simulink model "text28"  (R2014a)
settings: Solver=FixedStepDiscrete  StartTime=0.0  StopTime=10.0  FixedStep=0.0005  RelTol=1e-3
libraries: simulink x70, ec55xxlib x61
(part 3 of 3)

== system text28/驱动系统/驱动逻辑/油门规则/油门刹车冲突 ==
  油门 : Inport
  刹车 : Inport  Port=2
  反馈 : Inport  Port=3
  If : If  NumInputs=2  IfExpression=u1>25&u2==1
  Merge2 : Merge
  故障 : Subsystem  TreatAsAtomicUnit=on
  "正常  " : Subsystem  TreatAsAtomicUnit=on
  Out1 : Outport
  wires:
  If/1 -> 故障/Action
  If/2 -> "正常  "/Action
  故障/1(Out1) -> Merge2/1
  Merge2/1 -> Out1/1
  "正常  "/1(Out1) -> Merge2/2
  反馈/1 -> "正常  "/1(In1)
  油门/1 -> If/1
  刹车/1 -> If/2

== system text28/驱动系统/驱动逻辑/油门规则/油门死区判断 ==
  In1 : Inport
  If1 : If  IfExpression=u1<5
  Merge : Merge
  油门大于5% : Subsystem  TreatAsAtomicUnit=on
  油门小于5% : Subsystem  TreatAsAtomicUnit=on
  Out1 : Outport
  wires:
  If1/1 -> 油门小于5%/Action
  If1/2 -> 油门大于5%/Action
  油门小于5%/1(Out1) -> Merge/1
  油门大于5%/1(Out1) -> Merge/2
  Merge/1 -> Out1/1
  In1/1 -> If1/1

== system text28/驱动系统/驱动逻辑/电机测速/Function-Call Subsystem4 ==
  In3 : Inport
  In1 : Inport  Port=2
  In2 : Inport  Port=3
  In4 : Inport  Port=4
  function : TriggerPort  TriggerType=function-call
  Terminator1 : Terminator
  Terminator2 : Terminator
  Terminator3 : Terminator
  "Out2 " : Outport
  wires:
  In3/1 -> Terminator2/1
  In1/1 -> Terminator1/1
  In2/1 -> "Out2 "/1
  In4/1 -> Terminator3/1

== system text28/驱动系统/驱动逻辑/电机测速/ReceiveMessages ==
  resive : Inport
  Active_Discharge_Enab_Ter : Terminator
  Data Type Conversion : DataTypeConversion
  Data Type Conversion1 : DataTypeConversion
  Gain : Gain  Gain=-1
  Gain1 : Gain  Gain=-1
  IGBT_Enable_Feedback_Ter : Terminator
  Livecounter_Ter : Terminator
  MeaModule : ec55xxlib/RapidECU_U2/11Calibration/MeaModule  signal=motor_speed
  MeaModule1 : ec55xxlib/RapidECU_U2/11Calibration/MeaModule  signal=motor_torque
  MotorACCurrent_Ter : Terminator
  Precharge_Allow_Ter : Terminator
  resive1 : Subsystem
  电机转速 : Outport
  电机扭矩 : Outport  Port=2
  wires:
  resive1/1(Precharge_Allow_Out) -> Precharge_Allow_Ter/1
  resive1/3(MotorACCurrent_Out) -> MotorACCurrent_Ter/1
  resive1/5(Livecounter_Out) -> Livecounter_Ter/1
  resive1/6(IGBT_Enable_Feedback_Out) -> IGBT_Enable_Feedback_Ter/1
  resive1/7(Active_Discharge_Enab_Out) -> Active_Discharge_Enab_Ter/1
  resive/1 -> resive1/1(input)
  MeaModule/1 -> 电机转速/1
  MeaModule1/1 -> 电机扭矩/1
  Gain/1 -> MeaModule/1
  resive1/4(Motor_Speed_Out) -> Data Type Conversion/1
  Data Type Conversion/1 -> Gain/1
  Gain1/1 -> MeaModule1/1
  resive1/2(MotorTorque_Out) -> Data Type Conversion1/1
  Data Type Conversion1/1 -> Gain1/1

== system text28/驱动系统/驱动逻辑/角度传感器/角度传感器数据处理及不可靠信号 ==
  角度1 : Inport
  角度2 : Inport  Port=2
  Abs : Abs
  Constant : Constant  Value=100
  MeaModule : ec55xxlib/RapidECU_U2/11Calibration/MeaModule  signal=apps_erro
  MeaModule1 : ec55xxlib/RapidECU_U2/11Calibration/MeaModule  signal=app_date1
  MeaModule3 : ec55xxlib/RapidECU_U2/11Calibration/MeaModule  signal=baifenbi3
  Product : Product
  Product1 : Product
  不可靠信号判断 : Subsystem
  油门数值处理 : Subsystem
  百分比转化 : Subsystem
  油门数值 : Outport
  油门百分比 : Outport  Port=2
  wires:
  Product/1 -> 油门数值/1
  角度2/1 -> 百分比转化/2(角度2), 油门数值处理/2(角度2)
  不可靠信号判断/1(Out1) -> MeaModule/1
  油门数值处理/1(油门数值) -> MeaModule1/1
  MeaModule/1 -> Product/2
  MeaModule1/1 -> Product/1
  百分比转化/1(Out2) -> Abs/1
  油门数值处理/2(油门百分比) -> 油门百分比/1
  角度1/1 -> 油门数值处理/1(角度1), 百分比转化/1(角度1)
  Abs/1 -> MeaModule3/1
  Constant/1 -> Product1/2
  Product1/1 -> 不可靠信号判断/1(In1)
  MeaModule3/1 -> Product1/1

== system text28/驱动系统/驱动逻辑/角度传感器/角度传感器是否正常 ==
  角度1 : Inport
  角度2 : Inport  Port=2
  If : If  NumInputs=2  IfExpression=u2 > 800 & u1>600 &u2 <2900&u1<2700
  If Action Subsystem : Subsystem  TreatAsAtomicUnit=on
  If Action Subsystem1 : Subsystem  TreatAsAtomicUnit=on
  Merge : Merge
  油门范围 : Outport
  wires:
  角度1/1 -> If/1
  If/1 -> If Action Subsystem1/Action
  If/2 -> If Action Subsystem/Action
  If Action Subsystem1/1(Out1) -> Merge/1
  If Action Subsystem/1(Out1) -> Merge/2
  Merge/1 -> 油门范围/1
  角度2/1 -> If/2

== system text28/驱动系统/驱动逻辑/制动与待驶/待驶激活/If Action Subsystem ==
  Action Port : ActionPort  ActionType=then
  Constant : Constant
  Out1 : Outport
  wires:
  Constant/1 -> Out1/1

== system text28/驱动系统/驱动逻辑/制动与待驶/待驶激活/If Action Subsystem1 ==
  Action Port : ActionPort  ActionType=else
  Constant : Constant  Value=0
  Out1 : Outport
  wires:
  Constant/1 -> Out1/1

== system text28/驱动系统/驱动逻辑/制动与待驶/待驶激活/If Action Subsystem2 ==
  Action Port : ActionPort  ActionType=then
  Constant : Constant
  Out1 : Outport
  wires:
  Constant/1 -> Out1/1

== system text28/驱动系统/驱动逻辑/制动与待驶/待驶激活/If Action Subsystem3 ==
  Action Port : ActionPort  ActionType=else
  Constant : Constant  Value=0
  Out1 : Outport
  wires:
  Constant/1 -> Out1/1

== system text28/驱动系统/驱动逻辑/制动与待驶/鸣笛1/If Action Subsystem ==
  Action Port : ActionPort  ActionType=then
  Constant2 : Constant
  Out1 : Outport
  wires:
  Constant2/1 -> Out1/1

== system text28/驱动系统/驱动逻辑/制动与待驶/鸣笛1/If Action Subsystem1 ==
  Action Port : ActionPort  ActionType=else
  Constant : Constant  Value=0
  Out1 : Outport
  wires:
  Constant/1 -> Out1/1

== system text28/驱动系统/驱动逻辑/制动与待驶/鸣笛1/鸣笛 ==
  In1 : Inport
  安全回路 : Inport  Port=2
  Constant3 : Constant
  Data Type Conversion : DataTypeConversion  OutDataTypeStr=uint32
  Data Type Conversion1 : DataTypeConversion  OutDataTypeStr=uint32
  If : If  IfExpression=u1>0&u1<150
  If Action Subsystem : Subsystem  TreatAsAtomicUnit=on
  If Action Subsystem1 : Subsystem  TreatAsAtomicUnit=on
  Merge : Merge
  Product : Product
  Sum : Sum  Inputs=|++
  Unit Delay : UnitDelay  SampleTime=-1
  蜂鸣器 : ec55xxlib/RapidECU_U2/06PowerDriverPWM/PowerDriverPWM  channel=117: O_PWM11_HS2A9  sampletime=-1
  wires:
  If/1 -> If Action Subsystem/Action
  Data Type Conversion/1 -> 蜂鸣器/1
  In1/1 -> Sum/1
  Data Type Conversion1/1 -> 蜂鸣器/2
  Constant3/1 -> Data Type Conversion/1
  If/2 -> If Action Subsystem1/Action
  Merge/1 -> Data Type Conversion1/1
  Product/1 -> Unit Delay/1, If/1
  Unit Delay/1 -> Sum/2
  If Action Subsystem/1(Out1) -> Merge/1
  If Action Subsystem1/1(Out1) -> Merge/2
  安全回路/1 -> Product/1
  Sum/1 -> Product/2

== system text28/驱动系统/驱动逻辑/油门规则/刹车判断/有刹车 ==
  Action Port : ActionPort  ActionType=else
  Constant : Constant  Value=0
  Out1 : Outport
  wires:
  Constant/1 -> Out1/1

== system text28/驱动系统/驱动逻辑/油门规则/刹车判断/没刹车 ==
  Action Port : ActionPort  ActionType=then
  Constant : Constant
  Out1 : Outport
  wires:
  Constant/1 -> Out1/1

== system text28/驱动系统/驱动逻辑/油门规则/动力允许判断/动力信号 ==
  Action Port : ActionPort  ActionType=then
  Constant : Constant
  Out1 : Outport
  wires:
  Constant/1 -> Out1/1

== system text28/驱动系统/驱动逻辑/油门规则/动力允许判断/故障信号 ==
  Action Port : ActionPort  ActionType=else
  Constant : Constant  Value=0
  Out1 : Outport
  wires:
  Constant/1 -> Out1/1

== system text28/驱动系统/驱动逻辑/油门规则/油门刹车冲突/故障 ==
  Action Port : ActionPort  ActionType=then
  Constant : Constant  Value=0
  Out1 : Outport
  wires:
  Constant/1 -> Out1/1

== system text28/驱动系统/驱动逻辑/油门规则/油门刹车冲突/正常   ==
  In1 : Inport
  Action Port : ActionPort  ActionType=else
  If : If  IfExpression=u1>=1
  Merge : Merge
  故障 : Subsystem  TreatAsAtomicUnit=on
  正常 : Subsystem  TreatAsAtomicUnit=on
  Out1 : Outport
  wires:
  In1/1 -> If/1
  If/1 -> 正常/Action
  If/2 -> 故障/Action
  正常/1(Out1) -> Merge/1
  故障/1(Out1) -> Merge/2
  Merge/1 -> Out1/1

== system text28/驱动系统/驱动逻辑/油门规则/油门死区判断/油门大于5% ==
  Action Port : ActionPort  ActionType=else
  Constant : Constant  Value=0
  Out1 : Outport
  wires:
  Constant/1 -> Out1/1

== system text28/驱动系统/驱动逻辑/油门规则/油门死区判断/油门小于5% ==
  Action Port : ActionPort  ActionType=then
  Constant : Constant
  Out1 : Outport
  wires:
  Constant/1 -> Out1/1

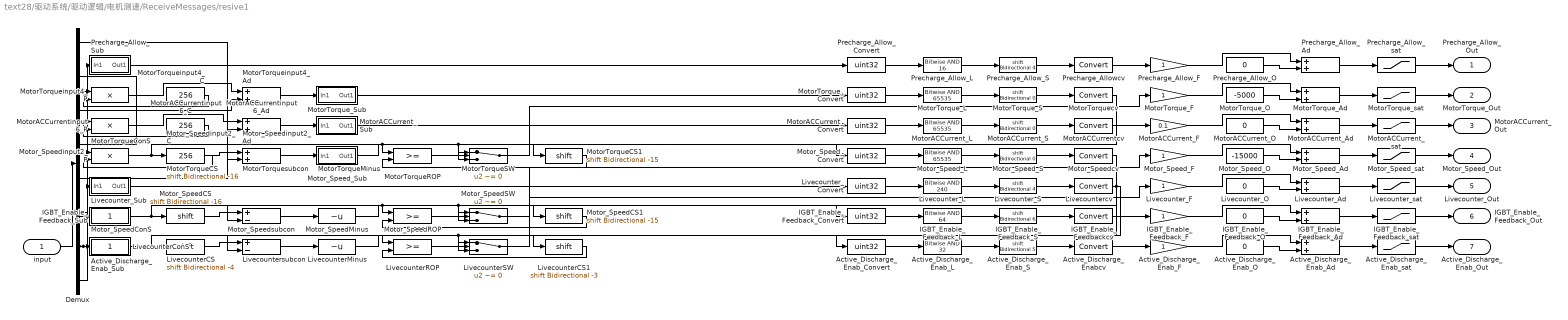
== system text28/驱动系统/驱动逻辑/电机测速/ReceiveMessages/resive1 ==
  input : Inport
  Active_Discharge_Enab_Ad : Sum
  Active_Discharge_Enab_Convert : DataTypeConversion  OutDataTypeStr=uint32
  Active_Discharge_Enab_F : Gain
  Active_Discharge_Enab_L : simulink/Logic and Bit Operations/Bitwise Operator  logicop=AND  UseBitMask=on  BitMask=32  BitMaskRealWorld=Stored Integer
  Active_Discharge_Enab_O : Constant  Value=0  OutDataTypeStr=single
  Active_Discharge_Enab_S : ArithShift  BitShiftNumber=5
  Active_Discharge_Enab_Sub : Subsystem
  Active_Discharge_Enab_sat : Saturate  UpperLimit=1  LowerLimit=0
  Active_Discharge_Enabcv : DataTypeConversion
  Demux : Demux  Outputs=8
  IGBT_Enable_Feedback_Ad : Sum
  IGBT_Enable_Feedback_Convert : DataTypeConversion  OutDataTypeStr=uint32
  IGBT_Enable_Feedback_F : Gain
  IGBT_Enable_Feedback_L : simulink/Logic and Bit Operations/Bitwise Operator  logicop=AND  UseBitMask=on  BitMask=64  BitMaskRealWorld=Stored Integer
  IGBT_Enable_Feedback_O : Constant  Value=0  OutDataTypeStr=single
  IGBT_Enable_Feedback_S : ArithShift  BitShiftNumber=6
  IGBT_Enable_Feedback_Sub : Subsystem
  IGBT_Enable_Feedback_sat : Saturate  UpperLimit=1  LowerLimit=0
  IGBT_Enable_Feedbackcv : DataTypeConversion
  LivecounterCS : ArithShift  BitShiftNumber=-4
  LivecounterCS1 : ArithShift  BitShiftNumber=-3
  LivecounterConS : Constant  OutDataTypeStr=single
  LivecounterMinus : UnaryMinus
  LivecounterROP : RelationalOperator  OutDataTypeStr=boolean
  LivecounterSW : Switch  Criteria=u2 ~= 0
  Livecounter_Ad : Sum
  Livecounter_Convert : DataTypeConversion  OutDataTypeStr=uint32
  Livecounter_F : Gain
  Livecounter_L : simulink/Logic and Bit Operations/Bitwise Operator  logicop=AND  UseBitMask=on  BitMask=240  BitMaskRealWorld=Stored Integer
  Livecounter_O : Constant  Value=0  OutDataTypeStr=single
  Livecounter_S : ArithShift  BitShiftNumber=4
  Livecounter_Sub : Subsystem
  Livecounter_sat : Saturate  UpperLimit=15  LowerLimit=0
  Livecountercv : DataTypeConversion
  Livecountersubcon : Sum  Inputs=+-
  MotorACCurrent_Ad : Sum
  MotorACCurrent_Convert : DataTypeConversion  OutDataTypeStr=uint32
  MotorACCurrent_F : Gain  Gain=0.1
  MotorACCurrent_L : simulink/Logic and Bit Operations/Bitwise Operator  logicop=AND  UseBitMask=on  BitMask=65535  BitMaskRealWorld=Stored Integer
  MotorACCurrent_O : Constant  Value=0  OutDataTypeStr=single
  MotorACCurrent_S : ArithShift
  MotorACCurrent_Sub : Subsystem
  MotorACCurrent_sat : Saturate  UpperLimit=1000  LowerLimit=0
  MotorACCurrentcv : DataTypeConversion
  MotorACCurrentinput6_Ad : Sum
  MotorACCurrentinput6_C : Constant  Value=256
  MotorACCurrentinput6_P : Product
  MotorTorqueCS : ArithShift  BitShiftNumber=-16
  MotorTorqueCS1 : ArithShift  BitShiftNumber=-15
  MotorTorqueConS : Constant  OutDataTypeStr=single
  MotorTorqueMinus : UnaryMinus
  MotorTorqueROP : RelationalOperator  OutDataTypeStr=boolean
  MotorTorqueSW : Switch  Criteria=u2 ~= 0
  MotorTorque_Ad : Sum
  MotorTorque_Convert : DataTypeConversion  OutDataTypeStr=uint32
  MotorTorque_F : Gain
  MotorTorque_L : simulink/Logic and Bit Operations/Bitwise Operator  logicop=AND  UseBitMask=on  BitMask=65535  BitMaskRealWorld=Stored Integer
  MotorTorque_O : Constant  Value=-5000  OutDataTypeStr=single
  MotorTorque_S : ArithShift
  MotorTorque_Sub : Subsystem
  MotorTorque_sat : Saturate  UpperLimit=5000  LowerLimit=-5000
  MotorTorquecv : DataTypeConversion
  MotorTorqueinput4_Ad : Sum
  MotorTorqueinput4_C : Constant  Value=256
  MotorTorqueinput4_P : Product
  MotorTorquesubcon : Sum  Inputs=+-
  Motor_SpeedCS : ArithShift  BitShiftNumber=-16
  Motor_SpeedCS1 : ArithShift  BitShiftNumber=-15
  Motor_SpeedConS : Constant  OutDataTypeStr=single
  Motor_SpeedMinus : UnaryMinus
  Motor_SpeedROP : RelationalOperator  OutDataTypeStr=boolean
  Motor_SpeedSW : Switch  Criteria=u2 ~= 0
  Motor_Speed_Ad : Sum
  Motor_Speed_Convert : DataTypeConversion  OutDataTypeStr=uint32
  Motor_Speed_F : Gain
  Motor_Speed_L : simulink/Logic and Bit Operations/Bitwise Operator  logicop=AND  UseBitMask=on  BitMask=65535  BitMaskRealWorld=Stored Integer
  Motor_Speed_O : Constant  Value=-15000  OutDataTypeStr=single
  Motor_Speed_S : ArithShift
  Motor_Speed_Sub : Subsystem
  Motor_Speed_sat : Saturate  UpperLimit=15000  LowerLimit=-15000
  Motor_Speedcv : DataTypeConversion
  Motor_Speedinput2_Ad : Sum
  Motor_Speedinput2_C : Constant  Value=256
  Motor_Speedinput2_P : Product
  Motor_Speedsubcon : Sum  Inputs=+-
  Precharge_Allow_Ad : Sum
  Precharge_Allow_Convert : DataTypeConversion  OutDataTypeStr=uint32
  Precharge_Allow_F : Gain
  Precharge_Allow_L : simulink/Logic and Bit Operations/Bitwise Operator  logicop=AND  UseBitMask=on  BitMask=16  BitMaskRealWorld=Stored Integer
  Precharge_Allow_O : Constant  Value=0  OutDataTypeStr=single
  Precharge_Allow_S : ArithShift  BitShiftNumber=4
  Precharge_Allow_Sub : Subsystem
  Precharge_Allow_sat : Saturate  UpperLimit=1  LowerLimit=0
  Precharge_Allowcv : DataTypeConversion
  Precharge_Allow_Out : Outport
  MotorTorque_Out : Outport  Port=2
  MotorACCurrent_Out : Outport  Port=3
  Motor_Speed_Out : Outport  Port=4
  Livecounter_Out : Outport  Port=5
  IGBT_Enable_Feedback_Out : Outport  Port=6
  Active_Discharge_Enab_Out : Outport  Port=7
  wires:
  Precharge_Allow_F/1 -> Precharge_Allow_Ad/1
  Precharge_Allow_O/1 -> Precharge_Allow_Ad/2
  Precharge_Allow_Ad/1 -> Precharge_Allow_sat/1
  Precharge_Allow_sat/1 -> Precharge_Allow_Out/1
  Demux/7 -> IGBT_Enable_Feedback_Sub/1(In1), Active_Discharge_Enab_Sub/1(In1), Precharge_Allow_Sub/1(In1)
  Precharge_Allow_Sub/1(Out1) -> Precharge_Allow_Convert/1
  Precharge_Allow_Convert/1 -> Precharge_Allow_L/1
  Precharge_Allow_L/1 -> Precharge_Allow_S/1
  Precharge_Allow_S/1 -> Precharge_Allowcv/1
  Precharge_Allowcv/1 -> Precharge_Allow_F/1
  MotorTorque_F/1 -> MotorTorque_Ad/1
  MotorTorque_O/1 -> MotorTorque_Ad/2
  MotorTorque_Ad/1 -> MotorTorque_sat/1
  MotorTorque_sat/1 -> MotorTorque_Out/1
  Demux/4 -> MotorTorqueinput4_P/1
  MotorTorqueinput4_C/1 -> MotorTorqueinput4_P/2
  MotorTorqueinput4_P/1 -> MotorTorqueinput4_Ad/1
  Demux/3 -> MotorTorqueinput4_Ad/2
  MotorTorqueinput4_Ad/1 -> MotorTorque_Sub/1(In1)
  MotorTorque_Sub/1(Out1) -> MotorTorque_Convert/1
  MotorTorque_Convert/1 -> MotorTorque_L/1
  MotorTorque_L/1 -> MotorTorque_S/1
  MotorTorque_S/1 -> MotorTorquecv/1
  MotorTorquecv/1 -> MotorTorqueROP/1, MotorTorquesubcon/2, MotorTorqueSW/3
  MotorTorqueConS/1 -> MotorTorqueCS/1, MotorTorqueCS1/1
  MotorTorqueCS1/1 -> MotorTorqueROP/2
  MotorTorqueCS/1 -> MotorTorquesubcon/1
  MotorTorquesubcon/1 -> MotorTorqueMinus/1
  MotorTorqueMinus/1 -> MotorTorqueSW/1
  MotorTorqueSW/1 -> MotorTorque_F/1
  MotorTorqueROP/1 -> MotorTorqueSW/2
  MotorACCurrent_F/1 -> MotorACCurrent_Ad/1
  MotorACCurrent_O/1 -> MotorACCurrent_Ad/2
  MotorACCurrent_Ad/1 -> MotorACCurrent_sat/1
  MotorACCurrent_sat/1 -> MotorACCurrent_Out/1
  Demux/6 -> MotorACCurrentinput6_P/1
  MotorACCurrentinput6_C/1 -> MotorACCurrentinput6_P/2
  MotorACCurrentinput6_P/1 -> MotorACCurrentinput6_Ad/1
  Demux/5 -> MotorACCurrentinput6_Ad/2
  MotorACCurrentinput6_Ad/1 -> MotorACCurrent_Sub/1(In1)
  MotorACCurrent_Sub/1(Out1) -> MotorACCurrent_Convert/1
  MotorACCurrent_Convert/1 -> MotorACCurrent_L/1
  MotorACCurrent_L/1 -> MotorACCurrent_S/1
  MotorACCurrent_S/1 -> MotorACCurrentcv/1
  MotorACCurrentcv/1 -> MotorACCurrent_F/1
  Motor_Speed_F/1 -> Motor_Speed_Ad/1
  Motor_Speed_O/1 -> Motor_Speed_Ad/2
  Motor_Speed_Ad/1 -> Motor_Speed_sat/1
  Motor_Speed_sat/1 -> Motor_Speed_Out/1
  Demux/2 -> Motor_Speedinput2_P/1
  Motor_Speedinput2_C/1 -> Motor_Speedinput2_P/2
  Motor_Speedinput2_P/1 -> Motor_Speedinput2_Ad/1
  Demux/1 -> Motor_Speedinput2_Ad/2
  Motor_Speedinput2_Ad/1 -> Motor_Speed_Sub/1(In1)
  Motor_Speed_Sub/1(Out1) -> Motor_Speed_Convert/1
  Motor_Speed_Convert/1 -> Motor_Speed_L/1
  Motor_Speed_L/1 -> Motor_Speed_S/1
  Motor_Speed_S/1 -> Motor_Speedcv/1
  Motor_Speedcv/1 -> Motor_SpeedROP/1, Motor_Speedsubcon/2, Motor_SpeedSW/3
  Motor_SpeedConS/1 -> Motor_SpeedCS/1, Motor_SpeedCS1/1
  Motor_SpeedCS1/1 -> Motor_SpeedROP/2
  Motor_SpeedCS/1 -> Motor_Speedsubcon/1
  Motor_Speedsubcon/1 -> Motor_SpeedMinus/1
  Motor_SpeedMinus/1 -> Motor_SpeedSW/1
  Motor_SpeedSW/1 -> Motor_Speed_F/1
  Motor_SpeedROP/1 -> Motor_SpeedSW/2
  Livecounter_F/1 -> Livecounter_Ad/1
  Livecounter_O/1 -> Livecounter_Ad/2
  Livecounter_Ad/1 -> Livecounter_sat/1
  Livecounter_sat/1 -> Livecounter_Out/1
  Demux/8 -> Livecounter_Sub/1(In1)
  Livecounter_Sub/1(Out1) -> Livecounter_Convert/1
  Livecounter_Convert/1 -> Livecounter_L/1
  Livecounter_L/1 -> Livecounter_S/1
  Livecounter_S/1 -> Livecountercv/1
  Livecountercv/1 -> Livecountersubcon/2, LivecounterSW/3, LivecounterROP/1
  LivecounterConS/1 -> LivecounterCS/1, LivecounterCS1/1
  LivecounterCS1/1 -> LivecounterROP/2
  LivecounterCS/1 -> Livecountersubcon/1
  Livecountersubcon/1 -> LivecounterMinus/1
  LivecounterMinus/1 -> LivecounterSW/1
  LivecounterSW/1 -> Livecounter_F/1
  LivecounterROP/1 -> LivecounterSW/2
  IGBT_Enable_Feedback_F/1 -> IGBT_Enable_Feedback_Ad/1
  IGBT_Enable_Feedback_O/1 -> IGBT_Enable_Feedback_Ad/2
  IGBT_Enable_Feedback_Ad/1 -> IGBT_Enable_Feedback_sat/1
  IGBT_Enable_Feedback_sat/1 -> IGBT_Enable_Feedback_Out/1
  IGBT_Enable_Feedback_Sub/1(Out1) -> IGBT_Enable_Feedback_Convert/1
  IGBT_Enable_Feedback_Convert/1 -> IGBT_Enable_Feedback_L/1
  IGBT_Enable_Feedback_L/1 -> IGBT_Enable_Feedback_S/1
  IGBT_Enable_Feedback_S/1 -> IGBT_Enable_Feedbackcv/1
  IGBT_Enable_Feedbackcv/1 -> IGBT_Enable_Feedback_F/1
  Active_Discharge_Enab_F/1 -> Active_Discharge_Enab_Ad/1
  Active_Discharge_Enab_O/1 -> Active_Discharge_Enab_Ad/2
  Active_Discharge_Enab_Ad/1 -> Active_Discharge_Enab_sat/1
  Active_Discharge_Enab_sat/1 -> Active_Discharge_Enab_Out/1
  Active_Discharge_Enab_Sub/1(Out1) -> Active_Discharge_Enab_Convert/1
  Active_Discharge_Enab_Convert/1 -> Active_Discharge_Enab_L/1
  Active_Discharge_Enab_L/1 -> Active_Discharge_Enab_S/1
  Active_Discharge_Enab_S/1 -> Active_Discharge_Enabcv/1
  Active_Discharge_Enabcv/1 -> Active_Discharge_Enab_F/1
  input/1 -> Demux/1

== system text28/驱动系统/驱动逻辑/角度传感器/角度传感器数据处理及不可靠信号/不可靠信号判断 ==
  In1 : Inport
  If Action Subsystem8 : Subsystem  TreatAsAtomicUnit=on
  If Action Subsystem9 : Subsystem  TreatAsAtomicUnit=on
  If4 : If  IfExpression=u1 >10
  Merge4 : Merge
  Out1 : Outport
  wires:
  In1/1 -> If4/1
  If4/2 -> If Action Subsystem9/Action
  Merge4/1 -> Out1/1
  If4/1 -> If Action Subsystem8/Action
  If Action Subsystem8/1(Out1) -> Merge4/1
  If Action Subsystem9/1(Out1) -> Merge4/2

== system text28/驱动系统/驱动逻辑/角度传感器/角度传感器数据处理及不可靠信号/油门数值处理 ==
  角度1 : Inport
  角度2 : Inport  Port=2
  Abs : Abs
  Abs1 : Abs
  Add : Sum  Inputs=+-
  Constant1 : Constant  Value=850
  Constant10 : Constant  Value=6
  Constant11 : Constant  Value=0.00006358
  Constant2 : Constant  Value=970
  Constant3 : Constant  Value=20  SampleTime=-1
  Divide : Product  Inputs=*/
  Gain1 : Gain  Gain=100
  Gain10 : Gain  Gain=0.5
  Gain2 : Gain  Gain=1/88
  Gain3 : Gain  Gain=1/89.25
  MeaModule1 : ec55xxlib/RapidECU_U2/11Calibration/MeaModule  signal=app_baifenbi
  MeaModule2 : ec55xxlib/RapidECU_U2/11Calibration/MeaModule  signal=jiaodu1
  MeaModule3 : ec55xxlib/RapidECU_U2/11Calibration/MeaModule  signal=jiaodu2
  MeaModule4 : ec55xxlib/RapidECU_U2/11Calibration/MeaModule  signal=apple
  MeaModule5 : ec55xxlib/RapidECU_U2/11Calibration/MeaModule  signal=app_add2
  MeaModule6 : ec55xxlib/RapidECU_U2/11Calibration/MeaModule  signal=app_konghou
  Product : Product
  Sum1 : Sum  Inputs=+-
  Sum3 : Sum  Inputs=+-
  Sum6 : Sum
  "空量程 " : Subsystem
  阈值 : Subsystem
  阈值2 : Subsystem
  油门数值 : Outport
  油门百分比 : Outport  Port=2
  wires:
  Sum6/1 -> Gain10/1
  Gain10/1 -> MeaModule4/1
  Product/1 -> MeaModule6/1
  Constant11/1 -> Add/2
  "空量程 "/1(Out1) -> Product/2
  Add/1 -> MeaModule5/1
  Constant3/1 -> Divide/2
  MeaModule1/1 -> 油门百分比/1
  Divide/1 -> Gain1/1
  Gain1/1 -> 阈值2/1(In1)
  Gain2/1 -> Sum6/1
  Gain3/1 -> Sum6/2
  阈值/1(Out1) -> 油门数值/1
  阈值2/1(Out1) -> MeaModule1/1
  MeaModule4/1 -> "空量程 "/1(In1), Divide/1
  Constant1/1 -> Sum1/2
  Sum3/1 -> Abs/1
  Sum1/1 -> Abs1/1
  Abs/1 -> MeaModule3/1
  MeaModule3/1 -> Gain3/1
  MeaModule2/1 -> Gain2/1
  角度2/1 -> Sum3/1
  Constant2/1 -> Sum3/2
  Abs1/1 -> MeaModule2/1
  角度1/1 -> Sum1/1
  MeaModule5/1 -> 阈值/1(In1)
  Constant10/1 -> Product/1
  MeaModule6/1 -> Add/1

== system text28/驱动系统/驱动逻辑/角度传感器/角度传感器数据处理及不可靠信号/百分比转化 ==
  角度1 : Inport
  角度2 : Inport  Port=2
  MeaModule1 : ec55xxlib/RapidECU_U2/11Calibration/MeaModule  signal=baifenbi1
  MeaModule2 : ec55xxlib/RapidECU_U2/11Calibration/MeaModule  signal=baifenbi2
  Sum2 : Sum  Inputs=+-
  角度归零化百分比1 : Subsystem
  角度归零化百分比2 : Subsystem
  Out2 : Outport
  wires:
  角度2/1 -> 角度归零化百分比1/1(角度2)
  角度归零化百分比1/1(Out1) -> MeaModule2/1
  角度归零化百分比2/1(Out1) -> MeaModule1/1
  Sum2/1 -> Out2/1
  角度1/1 -> 角度归零化百分比2/1(角度1)
  MeaModule1/1 -> Sum2/1
  MeaModule2/1 -> Sum2/2

== system text28/驱动系统/驱动逻辑/角度传感器/角度传感器是否正常/If Action Subsystem ==
  Action Port : ActionPort  ActionType=else
  Constant : Constant  Value=0  SampleTime=-1
  Out1 : Outport
  wires:
  Constant/1 -> Out1/1

== system text28/驱动系统/驱动逻辑/角度传感器/角度传感器是否正常/If Action Subsystem1 ==
  Action Port : ActionPort  ActionType=then
  Constant : Constant  SampleTime=-1
  Out1 : Outport
  wires:
  Constant/1 -> Out1/1

== system text28/驱动系统/驱动逻辑/制动与待驶/鸣笛1/鸣笛/If Action Subsystem ==
  Action Port : ActionPort  ActionType=then
  Constant : Constant
  Out1 : Outport
  wires:
  Constant/1 -> Out1/1

== system text28/驱动系统/驱动逻辑/制动与待驶/鸣笛1/鸣笛/If Action Subsystem1 ==
  Action Port : ActionPort  ActionType=else
  Constant : Constant  Value=0
  Out1 : Outport
  wires:
  Constant/1 -> Out1/1

== system text28/驱动系统/驱动逻辑/油门规则/油门刹车冲突/正常  /故障 ==
  Action Port : ActionPort  ActionType=else
  Constant : Constant  Value=0
  Out1 : Outport
  wires:
  Constant/1 -> Out1/1

== system text28/驱动系统/驱动逻辑/油门规则/油门刹车冲突/正常  /正常 ==
  Action Port : ActionPort  ActionType=then
  Constant : Constant
  Out1 : Outport
  wires:
  Constant/1 -> Out1/1

== system text28/驱动系统/驱动逻辑/电机测速/ReceiveMessages/resive1/Active_Discharge_Enab_Sub ==
  In1 : Inport
  Out1 : Outport
  wires:
  In1/1 -> Out1/1

== system text28/驱动系统/驱动逻辑/电机测速/ReceiveMessages/resive1/IGBT_Enable_Feedback_Sub ==
  In1 : Inport
  Out1 : Outport
  wires:
  In1/1 -> Out1/1

== system text28/驱动系统/驱动逻辑/电机测速/ReceiveMessages/resive1/Livecounter_Sub ==
  In1 : Inport
  Out1 : Outport
  wires:
  In1/1 -> Out1/1

== system text28/驱动系统/驱动逻辑/电机测速/ReceiveMessages/resive1/MotorACCurrent_Sub ==
  In1 : Inport
  Out1 : Outport
  wires:
  In1/1 -> Out1/1

== system text28/驱动系统/驱动逻辑/电机测速/ReceiveMessages/resive1/MotorTorque_Sub ==
  In1 : Inport
  Out1 : Outport
  wires:
  In1/1 -> Out1/1

== system text28/驱动系统/驱动逻辑/电机测速/ReceiveMessages/resive1/Motor_Speed_Sub ==
  In1 : Inport
  Out1 : Outport
  wires:
  In1/1 -> Out1/1

== system text28/驱动系统/驱动逻辑/电机测速/ReceiveMessages/resive1/Precharge_Allow_Sub ==
  In1 : Inport
  Out1 : Outport
  wires:
  In1/1 -> Out1/1

== system text28/驱动系统/驱动逻辑/角度传感器/角度传感器数据处理及不可靠信号/不可靠信号判断/If Action Subsystem8 ==
  Action Port : ActionPort  ActionType=then
  Constant : Constant  Value=0  SampleTime=-1
  Out1 : Outport
  wires:
  Constant/1 -> Out1/1

== system text28/驱动系统/驱动逻辑/角度传感器/角度传感器数据处理及不可靠信号/不可靠信号判断/If Action Subsystem9 ==
  Action Port : ActionPort  ActionType=else
  Constant : Constant  SampleTime=-1
  Out1 : Outport
  wires:
  Constant/1 -> Out1/1

== system text28/驱动系统/驱动逻辑/角度传感器/角度传感器数据处理及不可靠信号/油门数值处理/空量程  ==
  In1 : Inport
  If : If  IfExpression=u1 >= 1
  If Action Subsystem : Subsystem  TreatAsAtomicUnit=on
  If Action Subsystem1 : Subsystem  TreatAsAtomicUnit=on
  Merge : Merge
  Out1 : Outport
  wires:
  In1/1 -> If Action Subsystem/1(In1), If/1
  If/1 -> If Action Subsystem/Action
  If/2 -> If Action Subsystem1/Action
  If Action Subsystem1/1(Out1) -> Merge/2
  If Action Subsystem/1(Out1) -> Merge/1
  Merge/1 -> Out1/1

== system text28/驱动系统/驱动逻辑/角度传感器/角度传感器数据处理及不可靠信号/油门数值处理/阈值 ==
  In1 : Inport
  If : If  IfExpression="u1 >=  1"
  If Action Subsystem : Subsystem  TreatAsAtomicUnit=on
  If Action Subsystem1 : Subsystem  TreatAsAtomicUnit=on
  Merge : Merge
  Out1 : Outport
  wires:
  Merge/1 -> Out1/1
  If Action Subsystem/1(Out1) -> Merge/1
  If Action Subsystem1/1(Out1) -> Merge/2
  If/2 -> If Action Subsystem1/Action
  If/1 -> If Action Subsystem/Action
  In1/1 -> If/1, If Action Subsystem/1(In1)

== system text28/驱动系统/驱动逻辑/角度传感器/角度传感器数据处理及不可靠信号/油门数值处理/阈值2 ==
  In1 : Inport
  If : If  IfExpression="u1 >=  0"
  If Action Subsystem : Subsystem  TreatAsAtomicUnit=on
  If Action Subsystem1 : Subsystem  TreatAsAtomicUnit=on
  Merge : Merge
  Out1 : Outport
  wires:
  In1/1 -> If Action Subsystem/1(In1), If/1
  If/1 -> If Action Subsystem/Action
  If/2 -> If Action Subsystem1/Action
  If Action Subsystem1/1(Out1) -> Merge/2
  If Action Subsystem/1(Out1) -> Merge/1
  Merge/1 -> Out1/1

== system text28/驱动系统/驱动逻辑/角度传感器/角度传感器数据处理及不可靠信号/百分比转化/角度归零化百分比1 ==
  角度2 : Inport
  Product : Product  Inputs=*/
  Sum1 : Sum  Inputs=|+-
  初始值1 : Constant  Value=960
  总值1 : Constant  Value=1800
  Out1 : Outport
  wires:
  Product/1 -> Out1/1
  Sum1/1 -> Product/1
  总值1/1 -> Product/2
  角度2/1 -> Sum1/1
  初始值1/1 -> Sum1/2

== system text28/驱动系统/驱动逻辑/角度传感器/角度传感器数据处理及不可靠信号/百分比转化/角度归零化百分比2 ==
  角度1 : Inport
  Product : Product  Inputs=*/
  Sum1 : Sum  Inputs=|+-
  初始值1 : Constant  Value=830
  总值1 : Constant  Value=1780
  Out1 : Outport
  wires:
  总值1/1 -> Product/2
  Product/1 -> Out1/1
  Sum1/1 -> Product/1
  初始值1/1 -> Sum1/2
  角度1/1 -> Sum1/1

== system text28/驱动系统/驱动逻辑/角度传感器/角度传感器数据处理及不可靠信号/油门数值处理/空量程 /If Action Subsystem ==
  In1 : Inport
  Action Port : ActionPort  ActionType=then
  Out1 : Outport
  wires:
  In1/1 -> Out1/1

== system text28/驱动系统/驱动逻辑/角度传感器/角度传感器数据处理及不可靠信号/油门数值处理/空量程 /If Action Subsystem1 ==
  Action Port : ActionPort  ActionType=else
  Constant : Constant  Value=0  SampleTime=-1
  Out1 : Outport
  wires:
  Constant/1 -> Out1/1

== system text28/驱动系统/驱动逻辑/角度传感器/角度传感器数据处理及不可靠信号/油门数值处理/阈值/If Action Subsystem ==
  In1 : Inport
  Action Port : ActionPort  ActionType=then
  Out1 : Outport
  wires:
  In1/1 -> Out1/1

== system text28/驱动系统/驱动逻辑/角度传感器/角度传感器数据处理及不可靠信号/油门数值处理/阈值/If Action Subsystem1 ==
  Action Port : ActionPort  ActionType=else
  Constant : Constant  Value=0  SampleTime=-1
  Out1 : Outport
  wires:
  Constant/1 -> Out1/1

== system text28/驱动系统/驱动逻辑/角度传感器/角度传感器数据处理及不可靠信号/油门数值处理/阈值2/If Action Subsystem ==
  In1 : Inport
  Action Port : ActionPort  ActionType=then
  Out1 : Outport
  wires:
  In1/1 -> Out1/1

== system text28/驱动系统/驱动逻辑/角度传感器/角度传感器数据处理及不可靠信号/油门数值处理/阈值2/If Action Subsystem1 ==
  Action Port : ActionPort  ActionType=else
  Constant : Constant  Value=0  SampleTime=-1
  Out1 : Outport
  wires:
  Constant/1 -> Out1/1

== matlab function text28/驱动系统/驱动逻辑/Drive_AEKF/aekf_comp ==
  data: T_base input; T_opt output; w_rpm input; Te_raw input
function T_opt = aekf_comp(T_base, w_rpm, Te_raw)
% Reduced-order AEKF + active damping (VCU 10 ms)
% 2026 FS rules: T12.9.12 released pedal -> 0 torque; T12.10.5 CAN stale 500 ms
persistent x1 x2 P11 P12 P22 lam bad_t good_t comp_g buf idx sum_nis ff_lp
persistent w_prev Te_prev stale_cnt
if isempty(x1)
    x1 = 0.0; x2 = 0.0;
    P11 = 100.0; P12 = 0.0; P22 = 25.0;
    lam = 0.98; bad_t = 0.0; good_t = 0.0; comp_g = 1.0;
    buf = zeros(10,1); idx = 1; sum_nis = 0.0; ff_lp = 0.0;
    w_prev = 0.0; Te_prev = 0.0; stale_cnt = 0;
end
Ts = 0.01; J = 0.003; B = 5.0e-4;
Q1 = 1.0e-3; Q2 = 1.0; R = 0.01;
lam_max = 0.98; lam_min = 0.85; gam = 3.841; aa = 0.5;
Pcap1 = 100.0; Pcap2 = 400.0;
Kd = 0.01; WFF = 2.0*pi*5.0; FFMAX = 6.0; RAW = 10.0;
w = w_rpm*(2.0*pi/60.0);
Te = Te_raw/RAW;
% stale CAN guard: no change for 50 cycles = 500 ms
if (w_rpm == w_prev) && (Te_raw == Te_prev)
    stale_cnt = stale_cnt + 1;
else
    stale_cnt = 0;
end
w_prev = w_rpm; Te_prev = Te_raw;
stale = stale_cnt >= 50;
if ~stale
    % predict
    f1 = (Te - x2 - B*x1)/J;
    x1p = x1 + Ts*f1; x2p = x2;
    F11 = 1.0 - Ts*B/J; F12 = -Ts/J; F22 = 1.0;
    Pp11 = F11*(F11*P11 + F12*P12) + F12*(F11*P12 + F12*P22) + Q1;
    Pp12 = F11*P12 + F12*P22;
    Pp22 = P22 + Q2;
    % innovation and NIS
    eps = w - x1p;
    S = Pp11 + R;
    nis = (eps*eps)/S;
    sum_nis = sum_nis - buf(idx) + nis;
    buf(idx) = nis;
    idx = idx + 1;
    if idx > 10
        idx = 1;
    end
    nb = sum_nis/10.0;
    % adaptive forgetting factor
    arg = aa*(nb - gam);
    if arg > 50.0
        arg = 50.0;
    elseif arg < -50.0
        arg = -50.0;
    end
    lam = lam_min + (lam_max - lam_min)/(1.0 + exp(arg));
    if nb > gam
        Pp11 = Pp11/lam; Pp12 = Pp12/lam; Pp22 = Pp22/lam;
    end
    if Pp11 > Pcap1
        Pp11 = Pcap1;
    end
    if Pp22 > Pcap2
        Pp22 = Pcap2;
    end
    S = Pp11 + R;
    K1 = Pp11/S; K2 = Pp12/S;
    x1 = x1p + K1*eps; x2 = x2p + K2*eps;
    % Joseph covariance update
    IK11 = 1.0 - K1; IK21 = -K2; IK22 = 1.0;
    A11 = IK11*Pp11; A12 = IK11*Pp12;
    A21 = IK21*Pp11 + Pp12; A22 = IK21*Pp12 + Pp22;
    P11 = A11*IK11 + (K1*K1)*R;
    P12 = A11*IK21 + A12*IK22 + K1*K2*R;
    P22 = A21*IK21 + A22*IK22 + (K2*K2)*R;
    % fault-safe: fade out after 20 ms, recover after 50 ms
    if nb > gam
        bad_t = bad_t + Ts; good_t = 0.0;
    else
        good_t = good_t + Ts;
        if good_t > 0.05
            bad_t = 0.0;
        end
    end
    if bad_t > 0.02
        tgt = 0.0;
    else
        tgt = 1.0;
    end
    comp_g = comp_g + (tgt - comp_g)*Ts/0.01;
    % feedforward: low-pass + limit + gate
    ff_lp = ff_lp + Ts*WFF*(x2 - ff_lp);
    ff = ff_lp;
    if ff > FFMAX
        ff = FFMAX;
    elseif ff < -FFMAX
        ff = -FFMAX;
    end
    ff = ff*comp_g;
    % active damping
    damp = Kd*x1;
else
    % CAN stale: freeze estimator, disable feedforward and damping
    ff = 0.0; damp = 0.0; comp_g = 0.0;
end
% compose command in raw units
T_opt = T_base + (ff - damp)*RAW;
% T12.9.12 / T12.9.8: released pedal or APPS fault -> zero drive torque
if T_base <= 0.0
    T_opt = 0.0;
elseif T_opt < 0.0
    T_opt = 0.0;
elseif T_opt > 5000.0
    T_opt = 5000.0;
end
end
